simulink model "simmodelnew"  (R2017b)
settings: Solver=ode1  StartTime=0.0  StopTime=5  FixedStep=0.0001  RelTol=1e-3
undefined symbols (not defined in the file): Model_626, Sensoray
libraries: sldrtlib x4, simulink x1
settings Model: Creator=pawestlu  LastModifiedBy=lyericl
settings RTWCC: SystemTargetFile=sldrt.tlc  TemplateMakefile=sldrt.tmf  Description=Simulink Desktop Real-Time  RTWCompilerOptimization=on
settings CodeAppCC: MaxIdLength=95
settings SimulinkDesktopRealTimeCC: TargetPreCompLibLocation=C:\Program Files\MATLAB\R2017b\toolbox\sldrt\lib\win64

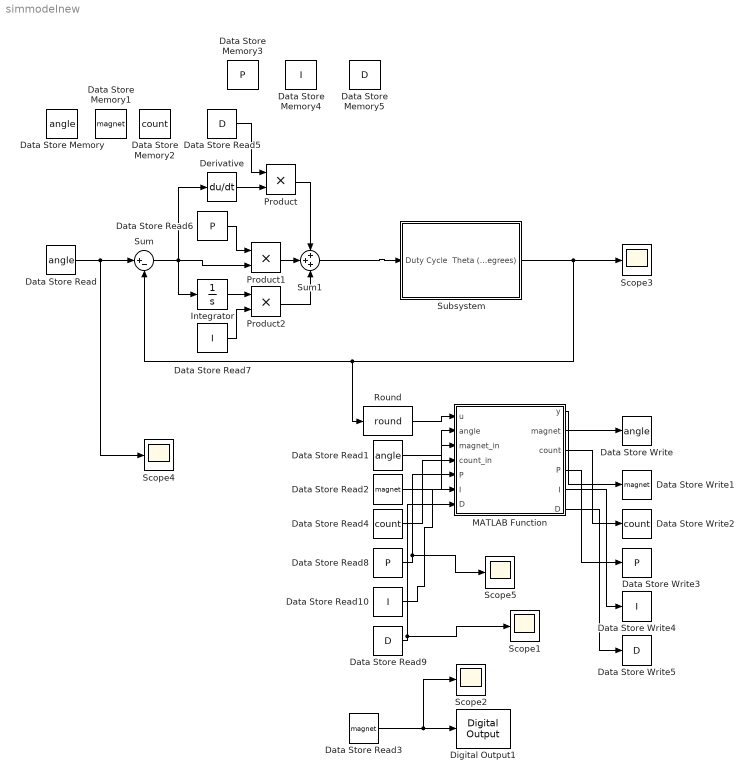
== system simmodelnew ==
  Data Store Memory : DataStoreMemory  DataStoreName=angle  ReadBeforeWriteMsg=warning  WriteAfterWriteMsg=warning  WriteAfterReadMsg=warning  InitialValue=90  ShowAdditionalParam=off
  Data Store Memory1 : DataStoreMemory  DataStoreName=magnet  ReadBeforeWriteMsg=warning  WriteAfterWriteMsg=warning  WriteAfterReadMsg=warning  InitialValue=5  ShowAdditionalParam=off
  Data Store Memory2 : DataStoreMemory  DataStoreName=count  ReadBeforeWriteMsg=warning  WriteAfterWriteMsg=warning  WriteAfterReadMsg=warning  ShowAdditionalParam=off
  Data Store Memory3 : DataStoreMemory  DataStoreName=P  ReadBeforeWriteMsg=warning  WriteAfterWriteMsg=warning  WriteAfterReadMsg=warning  InitialValue=2  ShowAdditionalParam=off
  Data Store Memory4 : DataStoreMemory  DataStoreName=I  ReadBeforeWriteMsg=warning  WriteAfterWriteMsg=warning  WriteAfterReadMsg=warning  ShowAdditionalParam=off
  Data Store Memory5 : DataStoreMemory  DataStoreName=D  ReadBeforeWriteMsg=warning  WriteAfterWriteMsg=warning  WriteAfterReadMsg=warning  InitialValue=0.2  ShowAdditionalParam=off
  Data Store Read : DataStoreRead  DataStoreName=angle
  Data Store Read1 : DataStoreRead  DataStoreName=angle
  Data Store Read10 : DataStoreRead  DataStoreName=I
  Data Store Read2 : DataStoreRead  DataStoreName=magnet
  Data Store Read3 : DataStoreRead  DataStoreName=magnet
  Data Store Read4 : DataStoreRead  DataStoreName=count
  Data Store Read5 : DataStoreRead  DataStoreName=D
  Data Store Read6 : DataStoreRead  DataStoreName=P
  Data Store Read7 : DataStoreRead  DataStoreName=I
  Data Store Read8 : DataStoreRead  DataStoreName=P
  Data Store Read9 : DataStoreRead  DataStoreName=D
  Data Store Write : DataStoreWrite  DataStoreName=angle
  Data Store Write1 : DataStoreWrite  DataStoreName=magnet
  Data Store Write2 : DataStoreWrite  DataStoreName=count
  Data Store Write3 : DataStoreWrite  DataStoreName=P
  Data Store Write4 : DataStoreWrite  DataStoreName=I
  Data Store Write5 : DataStoreWrite  DataStoreName=D
  Derivative : Derivative
  Digital Output1 : sldrtlib/Digital Output  SampleTime=0.0001  MaxMissedTicks=inf  ShowMissedTicks=off  YieldWhenWaiting=off  DrvName=Sensoray/Model_626  DrvAddress=4294967295  DrvOptions=zeros(1,0)  Channels=3  BitMode=1  InitialValue=5  FinalValue=5
      settings: AttributesFormatString=Sensoray\nModel 626 [auto]  SourceProductName=Simulink Desktop Real-Time  SourceProductBaseCode=WT
  Integrator : Integrator
  MATLAB Function : MATLAB Function  TreatAsAtomicUnit=on
  Product : Product
  Product1 : Product
  Product2 : Product
  Round : Rounding  Operator=round
  Scope{1..5} (5 alike) : Scope
  Subsystem : Subsystem
  Sum : Sum  Inputs=|+-
  Sum1 : Sum  Inputs=+++
  wires:
  Subsystem/1(Theta (degrees)) -> Scope3/1, Round/1, Sum/2
  Sum1/1 -> Subsystem/1(Duty Cycle)
  Sum/1 -> Product1/2, Derivative/1, Integrator/1
  Round/1 -> MATLAB Function/1(u)
  MATLAB Function/1(y) -> Data Store Write/1
  Data Store Read1/1 -> MATLAB Function/2(angle)
  Data Store Read2/1 -> MATLAB Function/3(magnet_in)
  MATLAB Function/2(magnet) -> Data Store Write1/1
  Data Store Read3/1 -> Scope2/1, Digital Output1/1
  Data Store Read4/1 -> MATLAB Function/4(count_in)
  MATLAB Function/3(count) -> Data Store Write2/1
  Derivative/1 -> Product/2
  Product/1 -> Sum1/1
  Data Store Read5/1 -> Product/1
  Product1/1 -> Sum1/2
  Data Store Read6/1 -> Product1/1
  Integrator/1 -> Product2/1
  Data Store Read7/1 -> Product2/2
  Product2/1 -> Sum1/3
  Data Store Read/1 -> Scope4/1, Sum/1
  Data Store Read8/1 -> Scope5/1, MATLAB Function/5("P ")
  Data Store Read10/1 -> MATLAB Function/6("I ")
  Data Store Read9/1 -> Scope1/1, MATLAB Function/7("D ")
  MATLAB Function/4(P) -> Data Store Write3/1
  MATLAB Function/5(I) -> Data Store Write4/1
  MATLAB Function/6(D) -> Data Store Write5/1

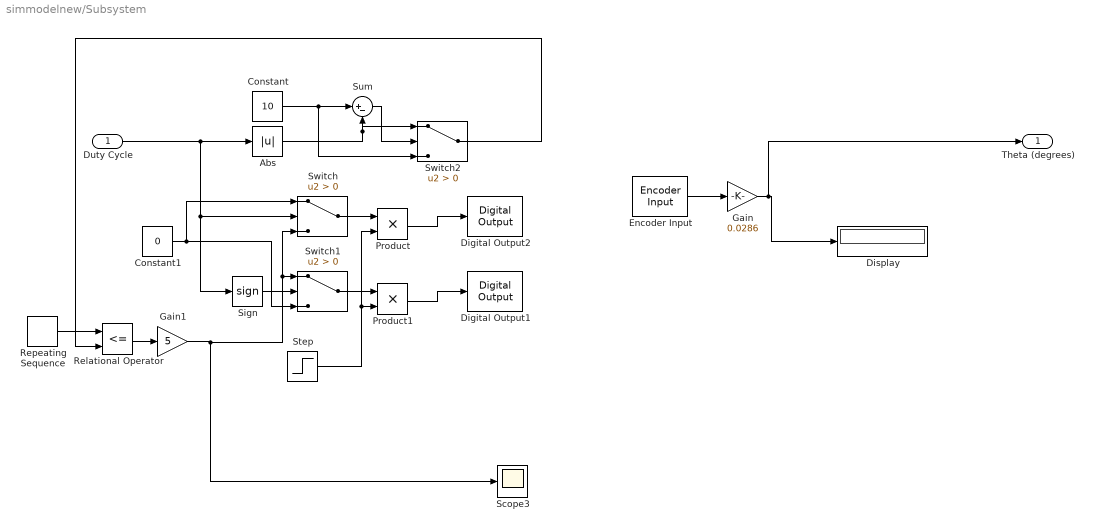
== system simmodelnew/Subsystem ==
  Duty Cycle : Inport
  Abs : Abs
  Constant : Constant  Value=10  SampleTime=0.0001
  Constant1 : Constant  Value=0  SampleTime=0.0001
  Digital Output1 : sldrtlib/Digital Output  SampleTime=0.0001  MaxMissedTicks=inf  ShowMissedTicks=off  YieldWhenWaiting=off  DrvName=Sensoray/Model_626  DrvAddress=4294967295  DrvOptions=zeros(1,0)  Channels=2  BitMode=1  InitialValue=[]  FinalValue=[]
      settings: AttributesFormatString=Sensoray\nModel 626 [auto]  SourceProductName=Simulink Desktop Real-Time  SourceProductBaseCode=WT
  Digital Output2 : sldrtlib/Digital Output  SampleTime=0.0001  MaxMissedTicks=inf  ShowMissedTicks=off  YieldWhenWaiting=off  DrvName=Sensoray/Model_626  DrvAddress=4294967295  DrvOptions=zeros(1,0)  Channels=1  BitMode=1  InitialValue=[]  FinalValue=[]
      settings: AttributesFormatString=Sensoray\nModel 626 [auto]  SourceProductName=Simulink Desktop Real-Time  SourceProductBaseCode=WT
  Display : Display
  Encoder Input : sldrtlib/Encoder Input  SampleTime=0.0001  MaxMissedTicks=inf  ShowMissedTicks=off  YieldWhenWaiting=off  DrvName=Sensoray/Model_626  DrvAddress=4294967295  DrvOptions=zeros(1,0)  Channels=1  QuadMode=3  IndexPulse=2  InputFilter=Inf  DataType=1
      settings: AttributesFormatString=Sensoray\nModel 626 [auto]  SourceProductName=Simulink Desktop Real-Time
  Gain : Gain  Gain=0.0286
  Gain1 : Gain  Gain=5
  Product : Product
  Product1 : Product
  Relational Operator : RelationalOperator  Operator=<=  OutDataTypeStr=boolean  RndMeth=Simplest
  Repeating Sequence : simulink/Sources/Repeating Sequence  rep_seq_t=[0 0.01]  rep_seq_y=[0 1]
  Scope3 : Scope
  Sign : Signum
  Step : Step  Time=4.9999  Before=1  After=0  SampleTime=0.0001
  Sum : Sum  Inputs=|+-
  Switch : Switch  Criteria=u2 > Threshold
  Switch1 : Switch  Criteria=u2 > Threshold
  Switch2 : Switch  Criteria=u2 > Threshold
  Theta (degrees) : Outport
  wires:
  Encoder Input/1 -> Gain/1
  Gain/1 -> Theta (degrees)/1, Display/1
  Duty Cycle/1 -> Sign/1, Switch/2, Abs/1
  Sign/1 -> Switch1/2
  Abs/1 -> Switch2/1, Sum/2
  Constant/1 -> Switch2/3, Sum/1
  Sum/1 -> Switch2/2
  Constant1/1 -> Switch1/3, Switch/1
  Switch1/1 -> Product1/1
  Switch/1 -> Product/1
  Product/1 -> Digital Output2/1
  Product1/1 -> Digital Output1/1
  Step/1 -> Product1/2, Product/2
  Repeating Sequence/1 -> Relational Operator/1
  Relational Operator/1 -> Gain1/1
  Switch2/1 -> Relational Operator/2
  Gain1/1 -> Switch/3, Switch1/1, Scope3/1

== matlab function simmodelnew/MATLAB Function ==
  data: u input; y output; angle input; magnet output; magnet_in input; count_in input; count output; P input; I input; D input; P output; I output; D output
function [y, magnet, count, P, I, D] = fcn(u, angle, magnet_in, count_in, P, I, D)
if u == 90 && angle == 90
    if(count_in == 4)
        y = 45;
        magnet = 0;
        count = 0;
        P = 6;
        I = 0.001;
        D = 3.8;
    else
        y = angle;
        magnet = 0;
        count = count_in + 1;
        P = 2;
        I = 0;
        D = 0.2;
    end
    
else if u == 45 && angle == 45
    y = 45;
    if(count_in == 1600)
        magnet = 5;
        count = count_in;
    else
        magnet = magnet_in;
        count = count_in + 1;
    end
else
    y = angle;
    magnet = magnet_in;
    count = count_in; 
end
end
